simulink model "Hydraulic_System"  (R2021b)
settings: Solver=VariableStepAuto  StartTime=0.0  StopTime=60  RelTol=1e-6
values from neighbouring files (symbols this model uses):
  A = 31.16e-4    (= 0.003116)    [Hydraulic_System_Parameters.m]
  a = 18.6e-4    (= 0.00186)    [Hydraulic_System_Parameters.m]
  beta = 10000    [Hydraulic_System_Parameters.m]
  D_P = 10.6e-6    (= 1.06e-05)    [Hydraulic_System_Parameters.m]
  FL = 40000    [Hydraulic_System_Parameters.m]
  k_EV = (32)/sqrt(22)    [Hydraulic_System_Parameters.m]
  k_RV = 500    [Hydraulic_System_Parameters.m]
  m1 = 650    [Hydraulic_System_Parameters.m]
  p_crackRV = 250    [Hydraulic_System_Parameters.m]
  V_pressure = 2.9444e-04    (= 0.00029444)    [Hydraulic_System_Parameters.m]
  xmax = 1.4    [Hydraulic_System_Parameters.m]
libraries: slpidlib x2
settings Model: Creator=shara  LastModifiedBy=rrai-HIL
settings SolverCC: ZeroCrossAlgorithm=Adaptive  AlgebraicLoopSolver=TrustRegion
settings DebuggingCC: MaskedZcDiagnostic=none  IgnoredZcDiagnostic=none  SFMachineParentedDataDiag=warning
settings ConfigComp: PLC_TargetIDE=codesys23  PLC_MultiTBSigbuilderTimeRange=off  PLC_InlineEnumCastFunction=off

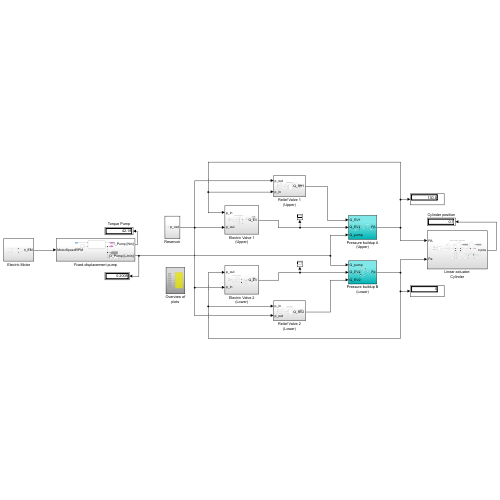
[thumbnail: Simulink's stored preview of the top-level diagram]
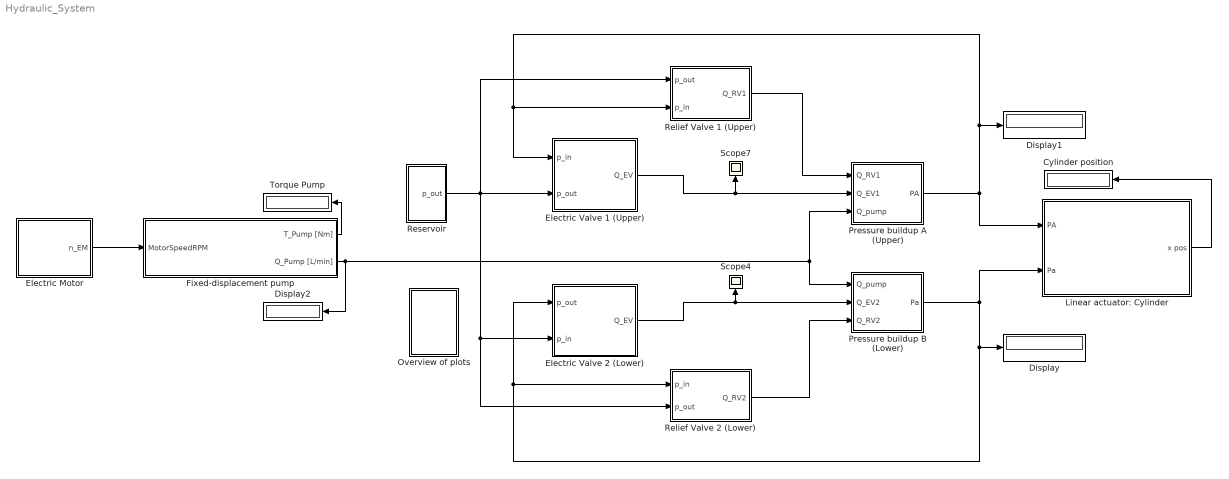
== system Hydraulic_System ==
  Cylinder position : Display
  Display : Display
  Display1 : Display
  Display2 : Display
  Electric Motor : Subsystem
  Electric Valve 1 (Upper) : Subsystem
  Electric Valve 2 (Lower) : Subsystem
  Fixed-displacement pump : Subsystem
  Linear actuator: Cylinder : Subsystem
  Overview of plots : Subsystem
  Pressure buildup A (Upper) : Subsystem
  Pressure buildup B (Lower) : Subsystem
  Relief Valve 1 (Upper) : Subsystem
  Relief Valve 2 (Lower) : Subsystem
  Reservoir : Subsystem
  Scope4 : Scope
  Scope7 : Scope
  Torque Pump : Display
  wires:
  Electric Motor/1(n_EM) -> Fixed-displacement pump/1(MotorSpeedRPM)
  Fixed-displacement pump/1(T_Pump [Nm]) -> Torque Pump/1
  Linear actuator: Cylinder/1(x pos) -> Cylinder position/1
  Pressure buildup A (Upper)/1(PA) -> Display1/1, Electric Valve 1 (Upper)/1(p_in), Relief Valve 1 (Upper)/2(p_in), Linear actuator: Cylinder/1(PA)
  Pressure buildup B (Lower)/1(Pa) -> Display/1, Electric Valve 2 (Lower)/1(p_out), Relief Valve 2 (Lower)/1(p_in), Linear actuator: Cylinder/2(Pa)
  Electric Valve 2 (Lower)/1(Q_EV) -> Pressure buildup B (Lower)/2(Q_EV2), Scope4/1
  Relief Valve 2 (Lower)/1(Q_RV2) -> Pressure buildup B (Lower)/3(Q_RV2)
  Relief Valve 1 (Upper)/1(Q_RV1) -> Pressure buildup A (Upper)/1(Q_RV1)
  Reservoir/1(p_out) -> Electric Valve 1 (Upper)/2(p_out), Relief Valve 1 (Upper)/1(p_out), Electric Valve 2 (Lower)/2(p_in), Relief Valve 2 (Lower)/2(p_out)
  Electric Valve 1 (Upper)/1(Q_EV) -> Pressure buildup A (Upper)/2(Q_EV1), Scope7/1
  Fixed-displacement pump/2(Q_Pump [L/min]) -> Display2/1, Pressure buildup A (Upper)/3(Q_pump), Pressure buildup B (Lower)/1(Q_pump)

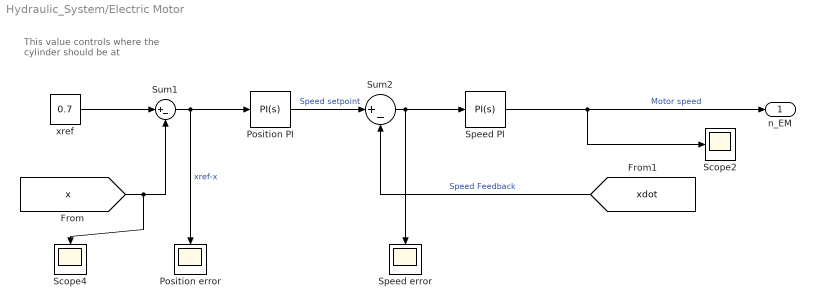
== system Hydraulic_System/Electric Motor ==
  note: This value controls
      | where the cylinder
      | should be at
  Position PI : slpidlib/PID Controller  Controller=PI  Form=Parallel  TimeDomain=Continuous-time  UseExternalTs=off  SampleTime=-1  IntegratorMethod=Forward Euler  FilterMethod=Forward Euler  ControllerParametersSource=internal  P=5  I=0.001  D=0  UseFilter=on  N=100  TunerSelectOption=Transfer Function Based (PID Tuner App)  InitialConditionSource=internal  InitialConditionForIntegrator=0  InitialConditionForFilter=0  DifferentiatorICPrevScaledInput=0  ExternalReset=none  TrackingMode=off  Kt=1  LimitOutput=on  SatLimitsSource=internal  UpperSaturationLimit=0.23  LowerSaturationLimit=-0.23  LinearizeAsGain=on  AntiWindupMode=none  Kb=1  POutMin=[]  POutMax=[]  IOutMin=[]  IOutMax=[]  DOutMin=[]  DOutMax=[]  NOutMin=[]  NOutMax=[]  SumOutMin=[]  SumOutMax=[]  SaturationOutMin=[]  SaturationOutMax=[]  PParamMin=[]  PParamMax=[]  IParamMin=[]  IParamMax=[]  DParamMin=[]  DParamMax=[]  NParamMin=[]  NParamMax=[]  KbParamMin=[]  KbParamMax=[]  KtParamMin=[]  KtParamMax=[]  KbOutMin=[]  KbOutMax=[]  KtOutMin=[]  KtOutMax=[]  IntegratorOutMin=[]  IntegratorOutMax=[]  FilterOutMin=[]  FilterOutMax=[]  SumI1OutMin=[]  SumI1OutMax=[]  SumI2OutMin=[]  SumI2OutMax=[]  SumI3OutMin=[]  SumI3OutMax=[]  SumI4OutMin=[]  SumI4OutMax=[]  SumDOutMin=[]  SumDOutMax=[]  DifferentiatorOutMin=[]  DifferentiatorOutMax=[]  FilterDiffOutCoefMin=[]  FilterDiffOutCoefMax=[]  ReciprocalOutMin=[]  ReciprocalOutMax=[]  SumDenOutMin=[]  SumDenOutMax=[]  SumNumOutMin=[]  SumNumOutMax=[]  DivideOutMin=[]  DivideOutMax=[]  UdiffTsProdOutMin=[]  UdiffTsProdOutMax=[]  NTsProdOutMin=[]  NTsProdOutMax=[]  UintegralTsProdOutMin=[]  UintegralTsProdOutMax=[]  UngainTsProdOutMin=[]  UngainTsProdOutMax=[]  IntegratorContinuousStateAttributes=''  IntegratorStateMustResolveToSignalObject=off  IntegratorRTWStateStorageClass=Auto  FilterContinuousStateAttributes=''  FilterStateMustResolveToSignalObject=off  FilterRTWStateStorageClass=Auto  ParallelPVariant=InternalParameters  IdealPVariant=Disabled  IVariant=InternalParameters  DVariant=Disabled  IntegratorVariant=Continuous  SatVariant=Enabled  AWVariant=Passthrough  PCopyVariant=Disabled  TRVariant=Disabled  FdbkBlocksVariant=Forward  IdealPFdbkVariant=Disabled  SatFdbkVariant=Disabled  DerivativeFilterVariant=Disabled  NVariant=Disabled  NCopyVariant=Disabled_SignalSpec  FilterICVariant=Disabled  IntegratorICVariant=InternalICs  ExternalResetVariant=Disabled  TRSumVariant=Passthrough  SumFdbkVariant=Disabled  SumVariant=Sum_PI  TsampFilterVariant=InternalTs  TsampNgainVariant=Passthrough  TsampIntegralVariant=Passthrough  ExternalSaturationOutDataTypeStr=Inherit: Same as second input
  Position error : Scope
  Scope2 : Scope
  Scope4 : Scope
  Speed PI : slpidlib/PID Controller  Controller=PI  Form=Parallel  TimeDomain=Continuous-time  UseExternalTs=off  SampleTime=-1  IntegratorMethod=Forward Euler  FilterMethod=Forward Euler  ControllerParametersSource=internal  P=2000  I=0.01  D=0  UseFilter=on  N=100  TunerSelectOption=Transfer Function Based (PID Tuner App)  InitialConditionSource=internal  InitialConditionForIntegrator=0  InitialConditionForFilter=0  DifferentiatorICPrevScaledInput=0  ExternalReset=none  TrackingMode=off  Kt=1  LimitOutput=off  SatLimitsSource=internal  UpperSaturationLimit=0.23  LowerSaturationLimit=-0.23  LinearizeAsGain=on  AntiWindupMode=none  Kb=1  POutMin=[]  POutMax=[]  IOutMin=[]  IOutMax=[]  DOutMin=[]  DOutMax=[]  NOutMin=[]  NOutMax=[]  SumOutMin=[]  SumOutMax=[]  SaturationOutMin=[]  SaturationOutMax=[]  PParamMin=[]  PParamMax=[]  IParamMin=[]  IParamMax=[]  DParamMin=[]  DParamMax=[]  NParamMin=[]  NParamMax=[]  KbParamMin=[]  KbParamMax=[]  KtParamMin=[]  KtParamMax=[]  KbOutMin=[]  KbOutMax=[]  KtOutMin=[]  KtOutMax=[]  IntegratorOutMin=[]  IntegratorOutMax=[]  FilterOutMin=[]  FilterOutMax=[]  SumI1OutMin=[]  SumI1OutMax=[]  SumI2OutMin=[]  SumI2OutMax=[]  SumI3OutMin=[]  SumI3OutMax=[]  SumI4OutMin=[]  SumI4OutMax=[]  SumDOutMin=[]  SumDOutMax=[]  DifferentiatorOutMin=[]  DifferentiatorOutMax=[]  FilterDiffOutCoefMin=[]  FilterDiffOutCoefMax=[]  ReciprocalOutMin=[]  ReciprocalOutMax=[]  SumDenOutMin=[]  SumDenOutMax=[]  SumNumOutMin=[]  SumNumOutMax=[]  DivideOutMin=[]  DivideOutMax=[]  UdiffTsProdOutMin=[]  UdiffTsProdOutMax=[]  NTsProdOutMin=[]  NTsProdOutMax=[]  UintegralTsProdOutMin=[]  UintegralTsProdOutMax=[]  UngainTsProdOutMin=[]  UngainTsProdOutMax=[]  IntegratorContinuousStateAttributes=''  IntegratorStateMustResolveToSignalObject=off  IntegratorRTWStateStorageClass=Auto  FilterContinuousStateAttributes=''  FilterStateMustResolveToSignalObject=off  FilterRTWStateStorageClass=Auto  ParallelPVariant=InternalParameters  IdealPVariant=Disabled  IVariant=InternalParameters  DVariant=Disabled  IntegratorVariant=Continuous  SatVariant=Disabled  AWVariant=Passthrough  PCopyVariant=Disabled  TRVariant=Disabled  FdbkBlocksVariant=Forward  IdealPFdbkVariant=Disabled  SatFdbkVariant=Disabled  DerivativeFilterVariant=Disabled  NVariant=Disabled  NCopyVariant=Disabled_SignalSpec  FilterICVariant=Disabled  IntegratorICVariant=InternalICs  ExternalResetVariant=Disabled  TRSumVariant=Passthrough  SumFdbkVariant=Disabled  SumVariant=Sum_PI  TsampFilterVariant=InternalTs  TsampNgainVariant=Passthrough  TsampIntegralVariant=Passthrough  ExternalSaturationOutDataTypeStr=Inherit: Same as second input
  Speed error : Scope
  Sum1 : Sum  Inputs=|+-
  Sum2 : Sum  Inputs=|+-
  xref : Constant  Value=0.7
  n_EM : Outport
  wires:
  Sum2/1 -> Speed PI/1, Speed error/1
  xref/1 -> Sum1/1
  Position PI/1 -> Sum2/1  "Speed setpoint"
  Speed PI/1 -> Scope2/1, n_EM/1  "Motor speed"
  Sum1/1 -> Position PI/1, Position error/1  "xref-x"
  [x] -> Sum1/2, Scope4/1
  [xdot] -> Sum2/2  "Speed Feedback"

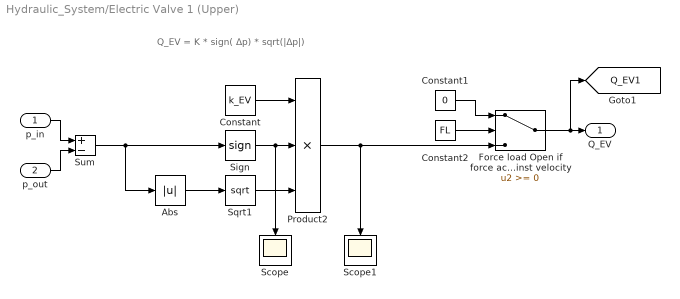
== system Hydraulic_System/Electric Valve 1 (Upper) ==
  note: Q_EV = K * sign( Δp) * sqrt(|Δp|)
  p_in : Inport
  p_out : Inport  Port=2
  Abs : Abs
  Constant : Constant  Value=k_EV
  Constant1 : Constant  Value=0
  Constant2 : Constant  Value=FL
  Force load Open if force acts against velocity : Switch
  Product2 : Product  Inputs=3
  Scope : Scope
  Scope1 : Scope
  Sign : Signum
  Sqrt1 : Sqrt  SaturateOnIntegerOverflow=on
  Sum : Sum  Inputs=+|-
  Q_EV : Outport
  tag scope: Q_EV1=global
  wires:
  Constant/1 -> Product2/1
  Sign/1 -> Product2/2, Scope/1
  Product2/1 -> Scope1/1, Force load Open if force acts against velocity/3
  Sqrt1/1 -> Product2/3
  Abs/1 -> Sqrt1/1
  p_in/1 -> Sum/1
  Sum/1 -> Sign/1, Abs/1
  p_out/1 -> Sum/2
  Force load Open if force acts against velocity/1 -> [Q_EV1], Q_EV/1
  Constant2/1 -> Force load Open if force acts against velocity/2
  Constant1/1 -> Force load Open if force acts against velocity/1

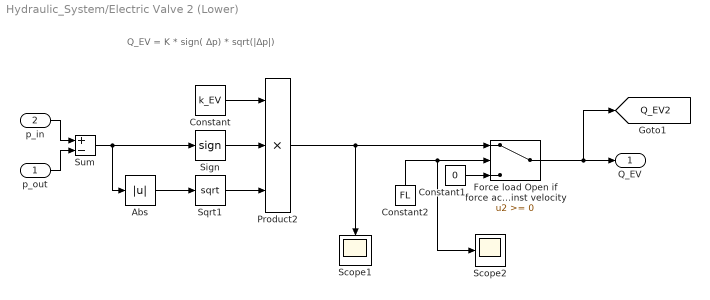
== system Hydraulic_System/Electric Valve 2 (Lower) ==
  note: Q_EV = K * sign( Δp) * sqrt(|Δp|)
  p_out : Inport
  p_in : Inport  Port=2
  Abs : Abs
  Constant : Constant  Value=k_EV
  Constant1 : Constant  Value=0
  Constant2 : Constant  Value=FL
  Force load Open if force acts against velocity : Switch
  Product2 : Product  Inputs=3
  Scope1 : Scope
  Scope2 : Scope
  Sign : Signum
  Sqrt1 : Sqrt  SaturateOnIntegerOverflow=on
  Sum : Sum  Inputs=+|-
  Q_EV : Outport
  tag scope: Q_EV2=global
  wires:
  Constant/1 -> Product2/1
  Sign/1 -> Product2/2
  Sqrt1/1 -> Product2/3
  Abs/1 -> Sqrt1/1
  p_in/1 -> Sum/1
  Sum/1 -> Abs/1, Sign/1
  p_out/1 -> Sum/2
  Constant1/1 -> Force load Open if force acts against velocity/3
  Product2/1 -> Force load Open if force acts against velocity/1, Scope1/1
  Force load Open if force acts against velocity/1 -> [Q_EV2], Q_EV/1
  Constant2/1 -> Scope2/1, Force load Open if force acts against velocity/2

== system Hydraulic_System/Fixed-displacement pump ==
  MotorSpeedRPM : Inport
  Display : Display
  Pump : Subsystem
  deltapMax : Constant  Value=250
  T_Pump [Nm] : Outport
  Q_Pump [L/min] : Outport  Port=2
  tag scope: Q_Pump=global
  wires:
  Pump/1(T_Pump [Nm]) -> T_Pump [Nm]/1
  deltapMax/1 -> Pump/2(deltapmax [bar])
  MotorSpeedRPM/1 -> Pump/1(n_EM [rev/min])
  Pump/2(Q_Pump [L/min]) -> Display/1, [Q_Pump], Q_Pump [L/min]/1

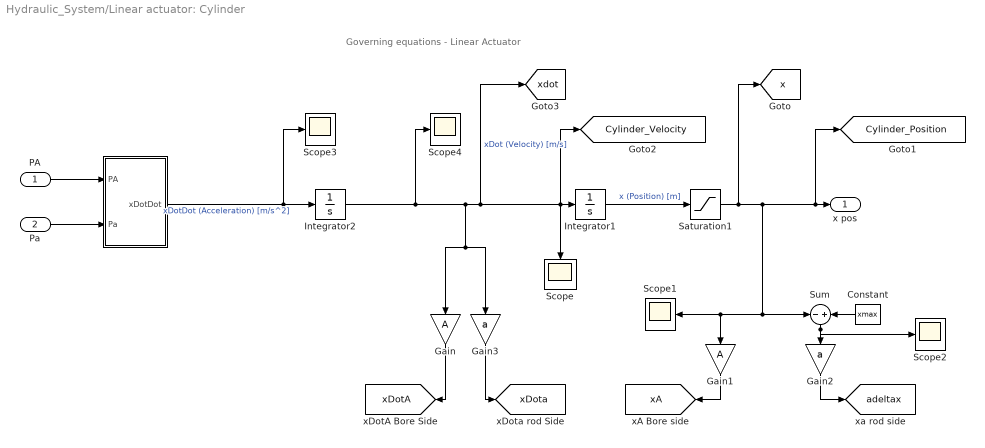
== system Hydraulic_System/Linear actuator: Cylinder ==
  note: Governing equations - Linear Actuator
  PA : Inport
  Pa : Inport  Port=2
  " " : Subsystem
  Constant : Constant  Value=xmax
  Gain : Gain  Gain=A
  Gain1 : Gain  Gain=A
  Gain2 : Gain  Gain=a
  Gain3 : Gain  Gain=a
  Integrator1 : Integrator
  Integrator2 : Integrator
  Saturation1 : Saturate  UpperLimit=0.7  LowerLimit=-0.7
  Scope{,1..4} (5 alike) : Scope
  Sum : Sum  Inputs=-|+
  x pos : Outport
  tag scope: Cylinder_Position=global, Cylinder_Velocity=global, adeltax=global, x=global, xA=global, xDotA=global, xDota=global, xdot=global
  wires:
  " "/1(xDotDot) -> Scope3/1, Integrator2/1  "xDotDot (Acceleration) [m/s^2]"
  Integrator2/1 -> [xdot], Scope/1, Integrator1/1, [Cylinder_Velocity], Gain/1, Gain3/1, Scope4/1  "xDot (Velocity) [m/s]"
  Integrator1/1 -> Saturation1/1  "x (Position) [m]"
  PA/1 -> " "/1(PA)
  Pa/1 -> " "/2(Pa)
  Gain/1 -> [xDotA]
  Gain1/1 -> [xA]
  Gain2/1 -> [adeltax]
  Gain3/1 -> [xDota]
  Sum/1 -> Scope2/1, Gain2/1
  Constant/1 -> Sum/2
  Saturation1/1 -> [x], Sum/1, Gain1/1, Scope1/1, [Cylinder_Position], x pos/1

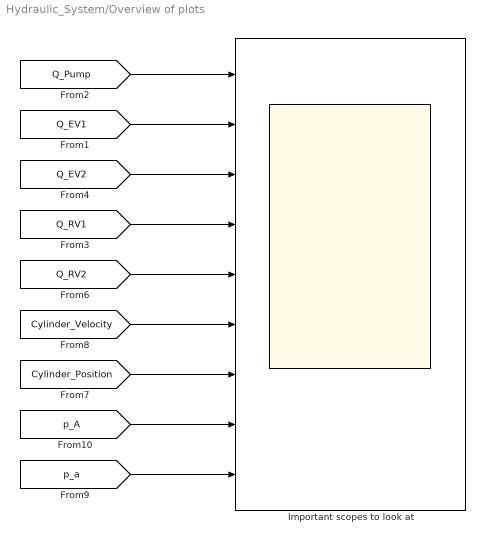
== system Hydraulic_System/Overview of plots ==
  Important scopes to look at : Scope  NumInputPorts=9
  wires:
  [Q_EV1] -> Important scopes to look at/2
  [Q_RV1] -> Important scopes to look at/4
  [Q_Pump] -> Important scopes to look at/1
  [Q_EV2] -> Important scopes to look at/3
  [Q_RV2] -> Important scopes to look at/5
  [Cylinder_Velocity] -> Important scopes to look at/6
  [Cylinder_Position] -> Important scopes to look at/7
  [p_A] -> Important scopes to look at/8
  [p_a] -> Important scopes to look at/9

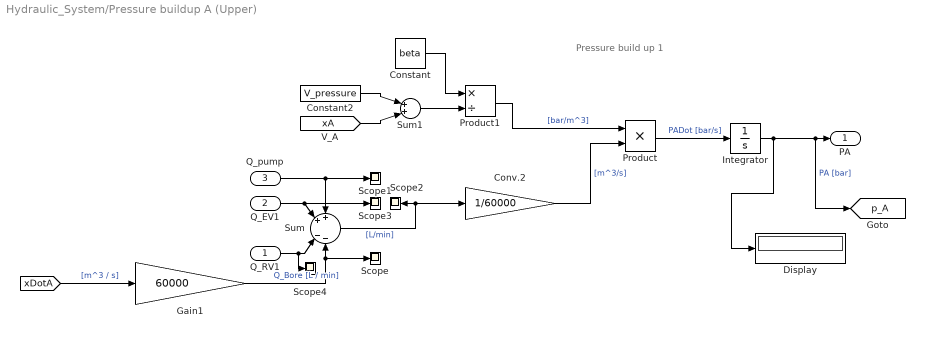
== system Hydraulic_System/Pressure buildup A (Upper) ==
  note: Pressure build up 1
  Q_RV1 : Inport
  Q_EV1 : Inport  Port=2
  Q_pump : Inport  Port=3
  Constant : Constant  Value=beta
  Constant2 : Constant  Value=V_pressure
  Conv.2 : Gain  Gain=1/60000
  Display : Display
  Gain1 : Gain  Gain=60000
  Integrator : Integrator
  Product : Product
  Product1 : Product  Inputs=*/
  Scope{,1..4} (5 alike) : Scope
  Sum : Sum  Inputs=++|--
  Sum1 : Sum  Inputs=|++|
  PA : Outport
  tag scope: p_A=global
  wires:
  Integrator/1 -> Display/1, [p_A], PA/1  "PA [bar]"
  Q_pump/1 -> Sum/1, Scope1/1
  Q_EV1/1 -> Scope3/1, Sum/2
  Q_RV1/1 -> Scope4/1, Sum/3
  Constant2/1 -> Sum1/1
  [xA] -> Sum1/2
  Product1/1 -> Product/1  "[bar/m^3]"
  Sum/1 -> Conv.2/1, Scope2/1  "[L/min]"
  Product/1 -> Integrator/1  "PADot [bar/s]"
  [xDotA] -> Gain1/1  "[m^3 / s]"
  Gain1/1 -> Sum/4, Scope/1  "Q_Bore [L / min]"
  Conv.2/1 -> Product/2  "[m^3/s]"
  Constant/1 -> Product1/1
  Sum1/1 -> Product1/2

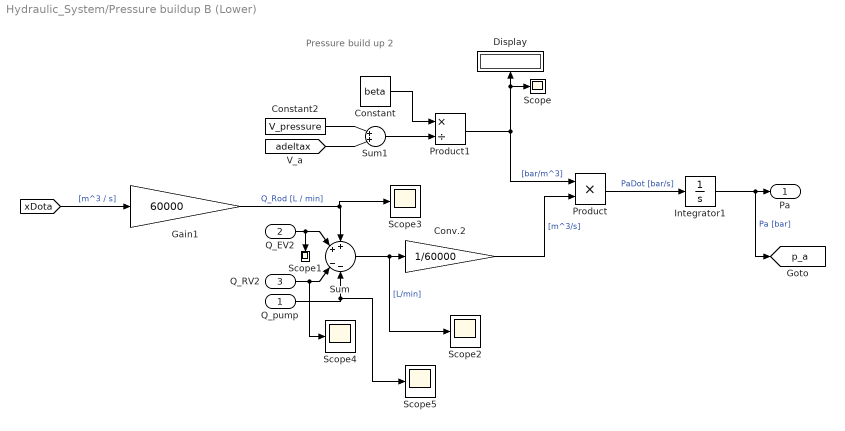
== system Hydraulic_System/Pressure buildup B (Lower) ==
  note: Pressure build up 2
  Q_pump : Inport
  Q_EV2 : Inport  Port=2
  Q_RV2 : Inport  Port=3
  Constant : Constant  Value=beta
  Constant2 : Constant  Value=V_pressure
  Conv.2 : Gain  Gain=1/60000
  Display : Display
  Gain1 : Gain  Gain=60000
  Integrator1 : Integrator
  Product : Product
  Product1 : Product  Inputs=*/
  Scope{,1..5} (6 alike) : Scope
  Sum : Sum  Inputs=++|--
  Sum1 : Sum  Inputs=|++|
  Pa : Outport
  tag scope: p_a=global
  wires:
  Product1/1 -> Display/1, Scope/1, Product/1  "[bar/m^3]"
  Constant2/1 -> Sum1/1
  Q_EV2/1 -> Sum/2, Scope1/1
  Sum/1 -> Scope2/1, Conv.2/1  "[L/min]"
  [adeltax] -> Sum1/2
  Q_RV2/1 -> Scope4/1, Sum/3
  Q_pump/1 -> Scope5/1, Sum/4
  Product/1 -> Integrator1/1  "PaDot [bar/s]"
  Integrator1/1 -> [p_a], Pa/1  "Pa [bar]"
  [xDota] -> Gain1/1  "[m^3 / s]"
  Gain1/1 -> Sum/1, Scope3/1  "Q_Rod [L / min]"
  Conv.2/1 -> Product/2  "[m^3/s]"
  Sum1/1 -> Product1/2
  Constant/1 -> Product1/1

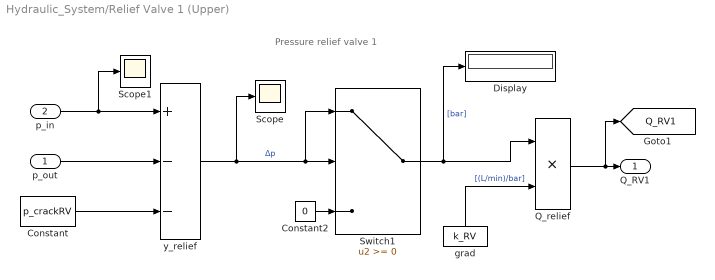
== system Hydraulic_System/Relief Valve 1 (Upper) ==
  note: Pressure relief valve 1
  p_out : Inport
  p_in : Inport  Port=2
  Constant : Constant  Value=p_crackRV
  Constant2 : Constant  Value=0
  Display : Display
  Q_relief : Product  RndMeth=Zero
  Scope : Scope
  Scope1 : Scope
  Switch1 : Switch
  grad : Constant  Value=k_RV
  y_relief : Sum  Inputs=+--
  Q_RV1 : Outport  VectorParamsAs1DForOutWhenUnconnected=off
  tag scope: Q_RV1=global
  wires:
  y_relief/1 -> Scope/1, Switch1/1, Switch1/2  "Δp"
  Switch1/1 -> Display/1, Q_relief/1  "[bar]"
  Q_relief/1 -> [Q_RV1], Q_RV1/1
  p_out/1 -> y_relief/2
  grad/1 -> Q_relief/2  "[(L/min)/bar]"
  Constant2/1 -> Switch1/3
  p_in/1 -> Scope1/1, y_relief/1
  Constant/1 -> y_relief/3

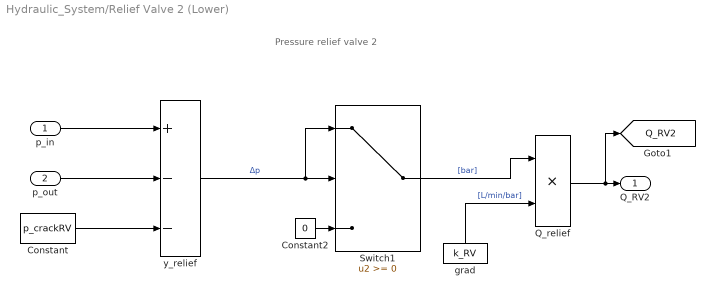
== system Hydraulic_System/Relief Valve 2 (Lower) ==
  note: Pressure relief valve 2
  p_in : Inport
  p_out : Inport  Port=2
  Constant : Constant  Value=p_crackRV
  Constant2 : Constant  Value=0
  Q_relief : Product  RndMeth=Zero
  Switch1 : Switch
  grad : Constant  Value=k_RV
  y_relief : Sum  Inputs=+--
  Q_RV2 : Outport  VectorParamsAs1DForOutWhenUnconnected=off
  tag scope: Q_RV2=global
  wires:
  Constant2/1 -> Switch1/3
  p_out/1 -> y_relief/2
  y_relief/1 -> Switch1/1, Switch1/2  "Δp"
  Switch1/1 -> Q_relief/1  "[bar]"
  p_in/1 -> y_relief/1
  grad/1 -> Q_relief/2  "[L/min/bar]"
  Constant/1 -> y_relief/3
  Q_relief/1 -> [Q_RV2], Q_RV2/1

== system Hydraulic_System/Reservoir ==
  Bar : Constant  Value=4
  p_out : Outport
  wires:
  Bar/1 -> p_out/1

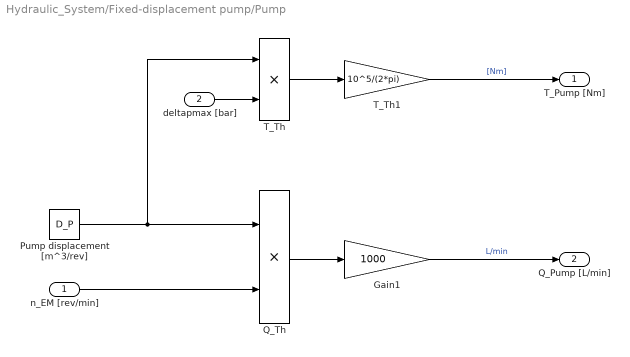
== system Hydraulic_System/Fixed-displacement pump/Pump ==
  n_EM [rev/min] : Inport
  deltapmax [bar] : Inport  Port=2
  Gain1 : Gain  Gain=1000
  Pump displacement [m^3/rev] : Constant  Value=D_P
  Q_Th : Product  RndMeth=Zero
  T_Th : Product  RndMeth=Zero
  T_Th1 : Gain  Gain=10^5/(2*pi)
  T_Pump [Nm] : Outport  VectorParamsAs1DForOutWhenUnconnected=off
  Q_Pump [L/min] : Outport  Port=2  VectorParamsAs1DForOutWhenUnconnected=off
  wires:
  Pump displacement [m^3/rev]/1 -> T_Th/1, Q_Th/1
  Q_Th/1 -> Gain1/1
  T_Th/1 -> T_Th1/1
  T_Th1/1 -> T_Pump [Nm]/1  "[Nm]"
  n_EM [rev/min]/1 -> Q_Th/2
  deltapmax [bar]/1 -> T_Th/2
  Gain1/1 -> Q_Pump [L/min]/1  "L/min"

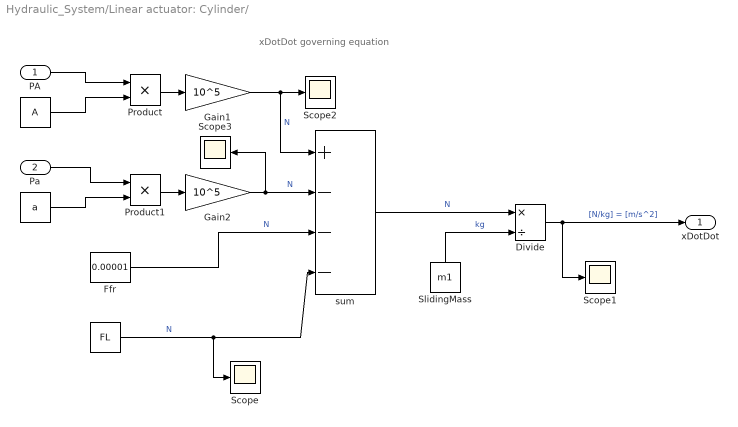
== system Hydraulic_System/Linear actuator: Cylinder/  ==
  note: xDotDot governing equation
  PA : Inport
  Pa : Inport  Port=2
  "   " : Constant  Value=A
  "    " : Constant  Value=a
  "      " : Constant  Value=FL
  "Divide " : Product  Inputs=*/
  Ffr : Constant  Value=0.00001
  Gain1 : Gain  Gain=10^5
  Gain2 : Gain  Gain=10^5
  Product : Product
  Product1 : Product
  Scope{,1..3} (4 alike) : Scope
  SlidingMass : Constant  Value=m1
  sum : Sum  Inputs=+---
  xDotDot : Outport
  wires:
  Ffr/1 -> sum/3  "N"
  "   "/1 -> Product/2
  "    "/1 -> Product1/2
  Pa/1 -> Product1/1
  PA/1 -> Product/1
  SlidingMass/1 -> "Divide "/2  "kg"
  sum/1 -> "Divide "/1  "N"
  "      "/1 -> sum/4, Scope/1  "N"
  Product1/1 -> Gain2/1
  Gain2/1 -> sum/2, Scope3/1  "N"
  Product/1 -> Gain1/1
  Gain1/1 -> Scope2/1, sum/1  "N"
  "Divide "/1 -> Scope1/1, xDotDot/1  "[N/kg] = [m/s^2]"
